simulink subsystem "pacejka"  (R2020b)
settings: Solver=VariableStepAuto  StartTime=0.0  StopTime=10.0  RelTol=1e-3
values from neighbouring files (symbols this model uses):
  Ax = 10    [main.m]
  Cd = 0.35    [main.m]
  d_air = 1.18    [main.m]
  Jf = (mtf*(Rt^2))/2    (= 30)    [main.m]
  Jr = (mtr*(Rt^2))/2    (= 120)    [main.m]
  M = 73000    [main.m]    (also in state_function.m)
  mu0 = 0.015    [main.m]
  mu1 = 7e-6    (= 7e-06)    [main.m]
  Rt = 0.5    [felt.m]    (also in k_pacejka.m; main.m)
  v0x = 70    [main.m]    (also in state_function.m)
settings Model: Creator=alema  LastModifiedBy=alema

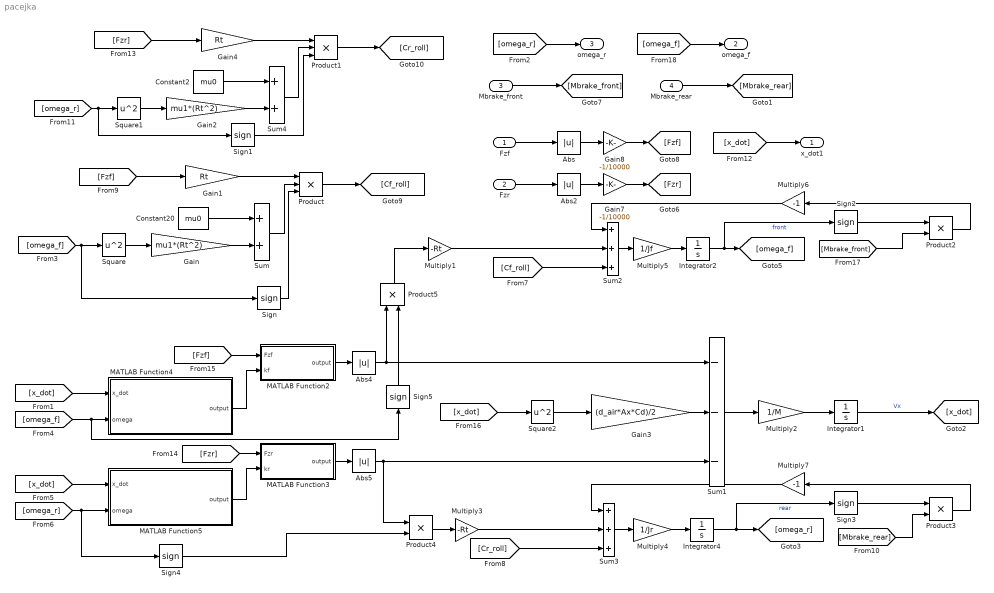
== system pacejka ==
  Fzf : Inport
  Fzr : Inport  Port=2
  Mbrake_front : Inport  Port=3
  Mbrake_rear : Inport  Port=4
  Abs{,2,4..5} (4 alike) : Abs
  Constant2 : Constant  Value=mu0
  Constant20 : Constant  Value=mu0
  Gain : Gain  Gain=mu1*(Rt^2)
  Gain1 : Gain  Gain=Rt
  Gain2 : Gain  Gain=mu1*(Rt^2)
  Gain3 : Gain  Gain=(d_air*Ax*Cd)/2
  Gain4 : Gain  Gain=Rt
  Gain7 : Gain  Gain=-1/10000
  Gain8 : Gain  Gain=-1/10000
  Integrator1 : Integrator  InitialCondition=v0x
  Integrator2 : Integrator  InitialCondition=-v0x/Rt
  Integrator4 : Integrator  InitialCondition=-v0x/Rt
  MATLAB Function2 : MATLAB Function  TreatAsAtomicUnit=on
  MATLAB Function3 : MATLAB Function  TreatAsAtomicUnit=on
  MATLAB Function4 : MATLAB Function  TreatAsAtomicUnit=on
  MATLAB Function5 : MATLAB Function  TreatAsAtomicUnit=on
  Multiply1 : Gain  Gain=-Rt
  Multiply2 : Gain  Gain=1/M
  Multiply3 : Gain  Gain=-Rt
  Multiply4 : Gain  Gain=1/Jr
  Multiply5 : Gain  Gain=1/Jf
  Multiply6 : Gain  Gain=-1
  Multiply7 : Gain  Gain=-1
  Product : Product  Inputs=3
  Product1 : Product  Inputs=3
  Product{2..5} (4 alike) : Product
  Sign{,1..5} (6 alike) : Signum
  Square : Math  Operator=square  SaturateOnIntegerOverflow=on
  Square1 : Math  Operator=square  SaturateOnIntegerOverflow=on
  Square2 : Math  Operator=square  SaturateOnIntegerOverflow=on
  Sum : Sum
  Sum1 : Sum  Inputs=---
  Sum2 : Sum  Inputs=+++
  Sum3 : Sum  Inputs=+++
  Sum4 : Sum
  x_dot1 : Outport
  omega_f : Outport  Port=2
  omega_r : Outport  Port=3
  wires:
  Sum1/1 -> Multiply2/1
  [omega_f] -> MATLAB Function4/2(omega), Sign5/1
  Multiply2/1 -> Integrator1/1
  Integrator1/1 -> [x_dot]  "Vx"
  Multiply5/1 -> Integrator2/1
  Multiply1/1 -> Sum2/2
  [Cf_roll] -> Sum2/3
  Sum2/1 -> Multiply5/1
  Gain3/1 -> Sum1/2
  Sum3/1 -> Multiply4/1
  Multiply3/1 -> Sum3/2
  Integrator4/1 -> [omega_r], Sign3/1  "rear"
  [Cr_roll] -> Sum3/3
  [x_dot] -> MATLAB Function4/1(x_dot)
  MATLAB Function5/1(output) -> MATLAB Function3/2(kr)
  [omega_r] -> MATLAB Function5/2(omega), Sign4/1
  Mbrake_front/1 -> [Mbrake_front]
  [omega_r] -> omega_r/1
  [omega_f] -> Square/1, Sign/1
  Square/1 -> Gain/1
  Gain/1 -> Sum/2
  Constant20/1 -> Sum/1
  [Fzf] -> Gain1/1
  Sum/1 -> Product/2
  Gain1/1 -> Product/1
  Square1/1 -> Gain2/1
  [omega_r] -> Square1/1, Sign1/1
  Gain4/1 -> Product1/1
  Gain2/1 -> Sum4/2
  Sum4/1 -> Product1/2
  Constant2/1 -> Sum4/1
  [Fzr] -> Gain4/1
  [Fzf] -> MATLAB Function2/1(Fzf)
  Fzf/1 -> Abs/1
  Abs/1 -> Gain8/1
  Fzr/1 -> Abs2/1
  Sign/1 -> Product/3
  Sign1/1 -> Product1/3
  MATLAB Function4/1(output) -> MATLAB Function2/2(kf)
  Gain8/1 -> [Fzf]
  Gain7/1 -> [Fzr]
  Abs2/1 -> Gain7/1
  Multiply4/1 -> Integrator4/1
  [Fzr] -> MATLAB Function3/1(Fzr)
  [x_dot] -> Square2/1
  Square2/1 -> Gain3/1
  Product1/1 -> [Cr_roll]
  Product/1 -> [Cf_roll]
  [x_dot] -> MATLAB Function5/1(x_dot)
  MATLAB Function2/1(output) -> Abs4/1
  MATLAB Function3/1(output) -> Abs5/1
  Integrator2/1 -> [omega_f], Sign2/1  "front"
  Sign2/1 -> Product2/1
  [Mbrake_front] -> Product2/2
  Product2/1 -> Multiply6/1
  [Mbrake_rear] -> Product3/2
  Product3/1 -> Multiply7/1
  Sign3/1 -> Product3/1
  Sign4/1 -> Product4/2
  Product4/1 -> Multiply3/1
  Product5/1 -> Multiply1/1
  Sign5/1 -> Product5/2
  Multiply6/1 -> Sum2/1
  Multiply7/1 -> Sum3/1
  Abs4/1 -> Product5/1, Sum1/1
  Abs5/1 -> Product4/1, Sum1/3
  Mbrake_rear/1 -> [Mbrake_rear]
  [x_dot] -> x_dot1/1
  [omega_f] -> omega_f/1

== matlab function pacejka/MATLAB Function2 ==
  data: Fzf input; output output; kf input
function output = function_f_pacejka(Fzf,kf)
    output=f_pacejka(Fzf,kf);
end

== matlab function pacejka/MATLAB Function3 ==
  data: Fzr input; output output; kr input
function output = function_f_pacejka(Fzr,kr)
    output=f_pacejka(Fzr,kr);
end

== matlab function pacejka/MATLAB Function4 ==
  data: x_dot input; output output; omega input
function output = function_k_pacejka(x_dot,omega)
    output=k_pacejka(x_dot,omega);
end

== matlab function pacejka/MATLAB Function5 ==
  data: x_dot input; output output; omega input
function output = function_k_pacejka(x_dot,omega)
    output=k_pacejka(x_dot,omega);
end
